simulink model "block_representation"  (R2024b)
settings: Solver=VariableStepAuto  StartTime=0.0  StopTime=5  RelTol=1e-3
undefined symbols (not defined in the file or in its folder): dspblkCoreblockFVToolHelper, gcbh
settings Model: Creator=Markus  LastModifiedBy=Markus
settings SolverCC: ZeroCrossAlgorithm=Adaptive
settings DebuggingCC: AlgebraicLoopMsg=none  IgnoredZcDiagnostic=none
settings HardwareCC: ProdHWDeviceType=AMD->x86-64 (Windows64)

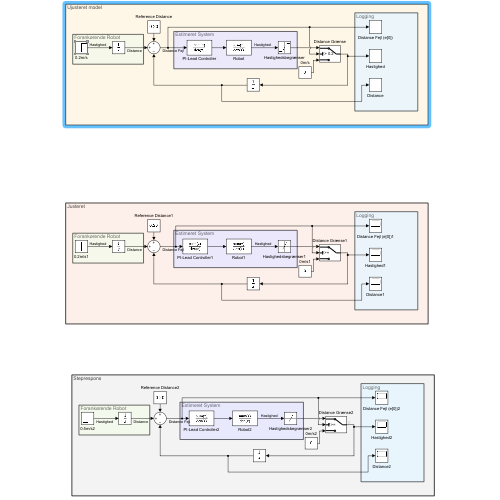
[thumbnail: Simulink's stored preview of the top-level diagram]
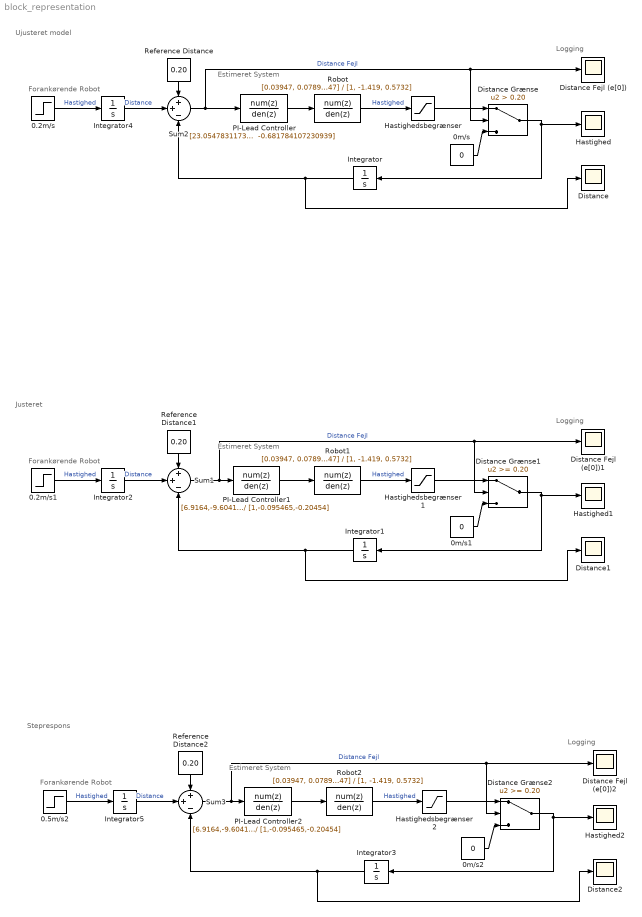
== system block_representation ==
  note: Ujusteret model
  note: Logging
  note: Forankørende Robot
  note: Estimeret System
  note: Justeret
  note: Forankørende Robot
  note: Logging
  note: Estimeret System
  note: Forankørende Robot
  note: Estimeret System
  note: Logging
  note: Steprespons
  0.2m/s : Step  Time=0  After=0.2  SampleTime=0
  0.2m/s1 : Step  Time=0  After=0.2  SampleTime=0  VectorParams1D=off
  0.5m/s2 : Step  Time=0  After=0.5  SampleTime=0  VectorParams1D=off
  0m/s : Constant  Value=0
  0m/s1 : Constant  Value=0
  0m/s2 : Constant  Value=0
  Distance : Scope
  Distance Fejl (e[0]) : Scope
  Distance Fejl (e[0])1 : Scope
  Distance Fejl (e[0])2 : Scope
  Distance Grænse : Switch  Criteria=u2 > Threshold  Threshold=0.20  SaturateOnIntegerOverflow=off  InputSameDT=off
  Distance Grænse1 : Switch  Threshold=0.20  SaturateOnIntegerOverflow=off  InputSameDT=off
  Distance Grænse2 : Switch  Threshold=0.20  SaturateOnIntegerOverflow=off  InputSameDT=off
  Distance1 : Scope
  Distance2 : Scope
  Hastighed : Scope
  Hastighed1 : Scope
  Hastighed2 : Scope
  Hastighedsbegrænser : Saturate  UpperLimit=0.4  LowerLimit=0  LinearizeAsGain=off
  Hastighedsbegrænser1 : Saturate  UpperLimit=0.4  LowerLimit=0  LinearizeAsGain=off
  Hastighedsbegrænser2 : Saturate  LowerLimit=0
  Integrator{,1..5} (6 alike) : Integrator
  PI-Lead Controller : DiscreteTransferFcn  LoadFcn=dspblkCoreblockFVToolHelper(gcbh,'load');  Numerator="[23.054783117344119 -32.013820463181034  11.070317218088730]"  Denominator="[1.000000000000000  -0.318215892769061  -0.681784107230939]"
      settings: CopyFcn=dspblkCoreblockFVToolHelper(gcbh,'copy');  DeleteFcn=dspblkCoreblockFVToolHelper(gcbh,'close');  ModelCloseFcn=dspblkCoreblockFVToolHelper(gcbh,'close');  PreSaveFcn=dspblkCoreblockFVToolHelper(gcbh,'presave');  PostSaveFcn=dspblkCoreblockFVToolHelper(gcbh,'postsave');  CloseFcn=dspblkCoreblockFVToolHelper(gcbh,'close');
  PI-Lead Controller1 : DiscreteTransferFcn  LoadFcn=dspblkCoreblockFVToolHelper(gcbh,'load');  Numerator=[6.9164,-9.6041,3.3211]  Denominator=[1,-0.095465,-0.20454]
      settings: CopyFcn=dspblkCoreblockFVToolHelper(gcbh,'copy');  DeleteFcn=dspblkCoreblockFVToolHelper(gcbh,'close');  ModelCloseFcn=dspblkCoreblockFVToolHelper(gcbh,'close');  PreSaveFcn=dspblkCoreblockFVToolHelper(gcbh,'presave');  PostSaveFcn=dspblkCoreblockFVToolHelper(gcbh,'postsave');  CloseFcn=dspblkCoreblockFVToolHelper(gcbh,'close');
  PI-Lead Controller2 : DiscreteTransferFcn  LoadFcn=dspblkCoreblockFVToolHelper(gcbh,'load');  Numerator=[6.9164,-9.6041,3.3211]  Denominator=[1,-0.095465,-0.20454]
      settings: CopyFcn=dspblkCoreblockFVToolHelper(gcbh,'copy');  DeleteFcn=dspblkCoreblockFVToolHelper(gcbh,'close');  ModelCloseFcn=dspblkCoreblockFVToolHelper(gcbh,'close');  PreSaveFcn=dspblkCoreblockFVToolHelper(gcbh,'presave');  PostSaveFcn=dspblkCoreblockFVToolHelper(gcbh,'postsave');  CloseFcn=dspblkCoreblockFVToolHelper(gcbh,'close');
  Reference Distance : Constant  Value=0.20
  Reference Distance1 : Constant  Value=0.20
  Reference Distance2 : Constant  Value=0.20
  Robot : DiscreteTransferFcn  LoadFcn=dspblkCoreblockFVToolHelper(gcbh,'load');  Numerator=[0.03947, 0.07894, 0.03947]  Denominator=[1, -1.419, 0.5732]
      settings: CopyFcn=dspblkCoreblockFVToolHelper(gcbh,'copy');  DeleteFcn=dspblkCoreblockFVToolHelper(gcbh,'close');  ModelCloseFcn=dspblkCoreblockFVToolHelper(gcbh,'close');  PreSaveFcn=dspblkCoreblockFVToolHelper(gcbh,'presave');  PostSaveFcn=dspblkCoreblockFVToolHelper(gcbh,'postsave');  CloseFcn=dspblkCoreblockFVToolHelper(gcbh,'close');
  Robot1 : DiscreteTransferFcn  LoadFcn=dspblkCoreblockFVToolHelper(gcbh,'load');  Numerator=[0.03947, 0.07894, 0.03947]  Denominator=[1, -1.419, 0.5732]
      settings: CopyFcn=dspblkCoreblockFVToolHelper(gcbh,'copy');  DeleteFcn=dspblkCoreblockFVToolHelper(gcbh,'close');  ModelCloseFcn=dspblkCoreblockFVToolHelper(gcbh,'close');  PreSaveFcn=dspblkCoreblockFVToolHelper(gcbh,'presave');  PostSaveFcn=dspblkCoreblockFVToolHelper(gcbh,'postsave');  CloseFcn=dspblkCoreblockFVToolHelper(gcbh,'close');
  Robot2 : DiscreteTransferFcn  LoadFcn=dspblkCoreblockFVToolHelper(gcbh,'load');  Numerator=[0.03947, 0.07894, 0.03947]  Denominator=[1, -1.419, 0.5732]
      settings: CopyFcn=dspblkCoreblockFVToolHelper(gcbh,'copy');  DeleteFcn=dspblkCoreblockFVToolHelper(gcbh,'close');  ModelCloseFcn=dspblkCoreblockFVToolHelper(gcbh,'close');  PreSaveFcn=dspblkCoreblockFVToolHelper(gcbh,'presave');  PostSaveFcn=dspblkCoreblockFVToolHelper(gcbh,'postsave');  CloseFcn=dspblkCoreblockFVToolHelper(gcbh,'close');
  Sum1 : Sum  Inputs=++-
  Sum2 : Sum  Inputs=++-
  Sum3 : Sum  Inputs=++-
  wires:
  Distance Grænse/1 -> Hastighed/1, Integrator/1
  0m/s/1 -> Distance Grænse/3
  0.2m/s/1 -> Integrator4/1  "Hastighed"
  Reference Distance/1 -> Sum2/1
  Robot/1 -> Hastighedsbegrænser/1  "Hastighed"
  Reference Distance1/1 -> Sum1/1
  Robot1/1 -> Hastighedsbegrænser1/1  "Hastighed"
  0m/s1/1 -> Distance Grænse1/3
  Distance Grænse1/1 -> Hastighed1/1, Integrator1/1
  0.2m/s1/1 -> Integrator2/1  "Hastighed"
  PI-Lead Controller/1 -> Robot/1
  Hastighedsbegrænser/1 -> Distance Grænse/1
  PI-Lead Controller1/1 -> Robot1/1
  Hastighedsbegrænser1/1 -> Distance Grænse1/1
  Integrator2/1 -> Sum1/2  "Distance"
  Sum1/1 -> Distance Grænse1/2, Distance Fejl (e[0])1/1, PI-Lead Controller1/1  "Distance Fejl"
  Sum2/1 -> PI-Lead Controller/1, Distance Grænse/2, Distance Fejl (e[0])/1  "Distance Fejl"
  Integrator4/1 -> Sum2/2  "Distance"
  Integrator1/1 -> Sum1/3, Distance1/1
  Integrator/1 -> Sum2/3, Distance/1
  0.5m/s2/1 -> Integrator5/1  "Hastighed"
  Sum3/1 -> Distance Grænse2/2, Distance Fejl (e[0])2/1, PI-Lead Controller2/1  "Distance Fejl"
  Hastighedsbegrænser2/1 -> Distance Grænse2/1
  PI-Lead Controller2/1 -> Robot2/1
  Integrator3/1 -> Sum3/3, Distance2/1
  Distance Grænse2/1 -> Hastighed2/1, Integrator3/1
  Reference Distance2/1 -> Sum3/1
  0m/s2/1 -> Distance Grænse2/3
  Robot2/1 -> Hastighedsbegrænser2/1  "Hastighed"
  Integrator5/1 -> Sum3/2  "Distance"
